simulink model "ex_lateral_dynamics"  (R2026a)
settings: Solver=VariableStepAuto
libraries: aerolibconvert2 x1
settings Model: Creator=doyeop  LastModifiedBy=doyeop

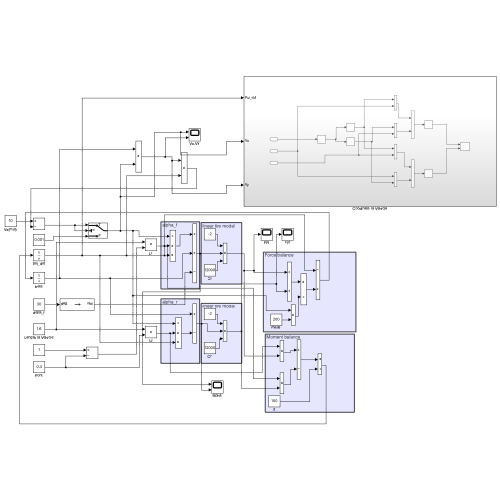
[thumbnail: Simulink's stored preview of the top-level diagram]
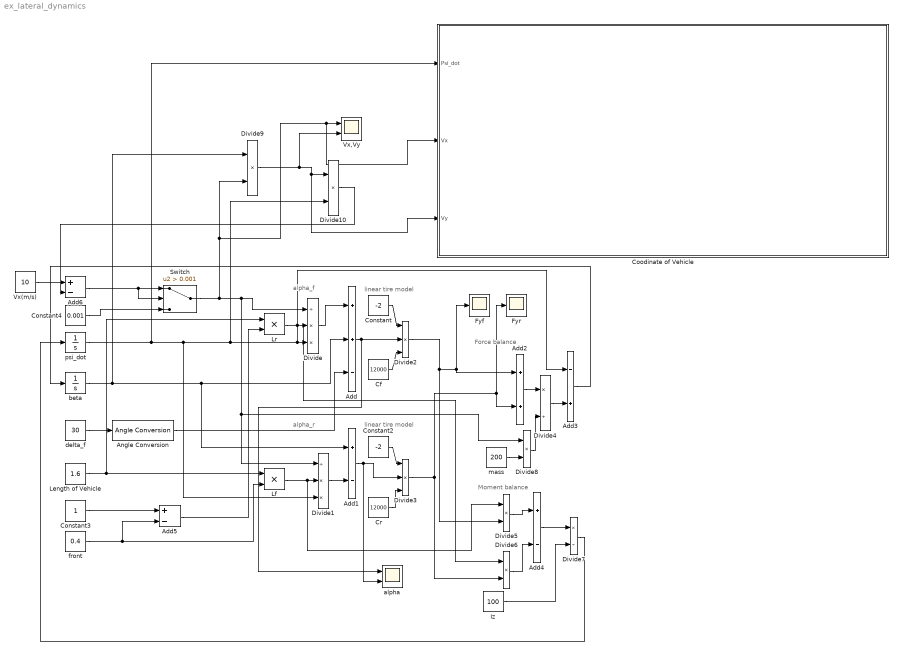
== system ex_lateral_dynamics ==
  note: linear tire model
  note: linear tire model
  note: alpha_f
  note: Moment balance
  note: alpha_r
  note: Force balance
  Add : Sum  Inputs=++-
  Add{1,4..6} (4 alike) : Sum  Inputs=+-
  Add2 : Sum
  Add3 : Sum  Inputs=-+
  Angle Conversion : aerolibconvert2/Angle Conversion  IU=deg  OU=rad
  Cf : Constant  Value=12000  SampleTime=-1
  Constant : Constant  Value=-2  SampleTime=-1
  Constant2 : Constant  Value=-2  SampleTime=-1
  Constant3 : Constant  SampleTime=-1
  Constant4 : Constant  Value=0.001
  Coodinate of Vehicle : Subsystem
  Cr : Constant  Value=12000  SampleTime=-1
  Divide : Product  Inputs=/**
  Divide1 : Product  Inputs=/**
  Divide{5..6,8..10} (5 alike) : Product  Inputs=**
  Divide2 : Product  Inputs=***
  Divide3 : Product  Inputs=***
  Divide4 : Product  Inputs=*/
  Divide7 : Product  Inputs=*/
  Fyf : Scope
      settings: ActiveDisplayYMinimum=-1407.4048741262529  ActiveDisplayYMaximum=11639.532558539519  DataLoggingVariableName=ScopeData14
  Fyr : Scope
      settings: ActiveDisplayYMinimum=-970.12534509010345  ActiveDisplayYMaximum=7745.6964021526865  DataLoggingVariableName=ScopeData15
  Iz : Constant  Value=100  SampleTime=-1
  Length of Vehicle : Constant  Value=1.6
  Lf : Product
  Lr : Product
  Switch : Switch  Criteria=u2 > Threshold  Threshold=0.001  SaturateOnIntegerOverflow=off  InputSameDT=off
  Vx(m/s) : Constant  Value=10
  Vx,Vy : Scope  NumInputPorts=2
      settings: ActiveDisplayYMinimum=-1.2499999999999998  ActiveDisplayYMaximum=11.25  DataLoggingVariableName=ScopeData16
  alpha : Scope  NumInputPorts=2
      settings: ActiveDisplayYMinimum=-0.10159314992994704  ActiveDisplayYMaximum=0.04167372337235864  DataLoggingVariableName=ScopeData27
  beta : Integrator
  delta_f : Constant  Value=30  SampleTime=-1
  front : Constant  Value=0.4  SampleTime=-1
  mass : Constant  Value=200
  psi_dot : Integrator
  wires:
  Cr/1 -> Divide3/3
  Add1/1 -> alpha/2, Divide3/2
  Constant2/1 -> Divide3/1
  Cf/1 -> Divide2/3
  Add3/1 -> beta/1
  Add/1 -> alpha/1, Divide2/2
  Constant/1 -> Divide2/1
  Divide10/1 -> Add6/2
  Angle Conversion/1 -> Add/3
  beta/1 -> Divide9/1, Add1/1, Add/2
  psi_dot/1 -> Add3/1, Divide/3, Divide10/2, Divide1/3, Coodinate of Vehicle/1(Psi_dot)
  Constant4/1 -> Switch/3
  Divide1/1 -> Add1/2
  Iz/1 -> Divide7/2
  Divide8/1 -> Divide4/2
  Switch/1 -> Divide1/1, Divide8/1, Divide/1, Divide9/2, Coodinate of Vehicle/2(Vx), Vx,Vy/1
  Divide/1 -> Add/1
  Divide9/1 -> Coodinate of Vehicle/3(Vy), Divide10/1, Vx,Vy/2
  Divide2/1 -> Divide5/2, Fyf/1, Add2/1
  Divide3/1 -> Add2/2, Fyr/1, Divide6/2
  Add2/1 -> Divide4/1
  delta_f/1 -> Angle Conversion/1
  mass/1 -> Divide8/2
  Divide7/1 -> psi_dot/1
  Add4/1 -> Divide7/1
  Divide6/1 -> Add4/2
  Divide5/1 -> Add4/1
  Divide4/1 -> Add3/2
  Add5/1 -> Lr/2
  Lf/1 -> Divide5/1, Divide1/2
  Lr/1 -> Divide6/1, Divide/2
  front/1 -> Lf/2, Add5/2
  Constant3/1 -> Add5/1
  Length of Vehicle/1 -> Lf/1, Lr/1
  Vx(m/s)/1 -> Add6/1
  Add6/1 -> Switch/2, Switch/1

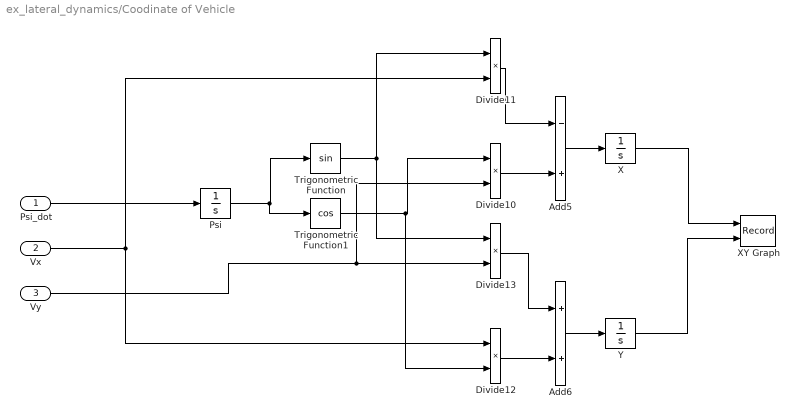
== system ex_lateral_dynamics/Coodinate of Vehicle ==
  Psi_dot : Inport
  Vx : Inport  Port=2
  Vy : Inport  Port=3
  Add5 : Sum  Inputs=-+
  Add6 : Sum
  Divide{10..13} (4 alike) : Product  Inputs=**
  Psi : Integrator
  Trigonometric Function : Trigonometry
  Trigonometric Function1 : Trigonometry  Operator=cos
  X : Integrator
  XY Graph : Record  NumPorts=2.0  FileSettingsInternal="{\"entries\":[{\"content\":{\"excelSettings\":{\"content\":{},\"type\":\"Streamout.ExcelSettings\"},\"parquetSettings\":{\"content\":{},\"type\":\"Streamout.ParquetSettings\"}},\"type\":\"Streamout.FileSettingStorage\",\"uuid\":\"\"}],\"packageUris\":[\"http:\\/\\/schema.mathworks.com\\/mf0\\/streamout_blocks\\/R2020a\"],\"version\":\"1.0\"}"  FrameSettings=[0, 0]  Layout=[1 1]  SignalsInternal="{\"entries\":[{\"content\":{\"signals\":[{\"content\":{\"blockPath\":[],\"dimensions\":[1],\"domain\":\"\",\"lineColor\":\"#a2142f\",\"plots\":[ 1 ],\"port\":1,\"sid\":[\"\"],\"signalID\":1,\"signalName\":\"X\"},\"type\":\"RecordBlkView.Signal\",\"uuid\":\"\"},{\"content\":{\"blockPath\":[],\"dimensions\":[1],\"domain\":\"\",\"lineColor\":\"#139fff\",\"plots\":[ 1 ],\"port\":2,\"sid\":[\"\"],\"signalID\":2,\"signalName\":\"Y\"},\"type\":\"RecordBlkView.Signal\",\"uuid\":\"\"}]},\"type\":\"RecordBlkView.InputSignals\",\"uuid\":\"\"}],\"packageUris\":[\"http:\\/\\/schema.mathworks.com\\/mf0\\/streamout_blocks\\/R2020a\"],\"version\":\"1.0\"}"  VisualizationBindings="{\"xyplotplugin\":{\"info\":[{\"series\":[{\"bindingParametersList\":[{\"parameter\":\"X-Axis\",\"signalID\":1,\"signalName\":\"X\"},{\"parameter\":\"Y-Axis\",\"signalID\":2,\"signalName\":\"Y\"}],\"seriesID\":0}],\"subplotID\":1}]}}"  CompatibilityTag=XY
  Y : Integrator
  wires:
  X/1 -> XY Graph/1
  Add6/1 -> Y/1
  Divide10/1 -> Add5/2
  Psi/1 -> Trigonometric Function1/1, Trigonometric Function/1
  Divide12/1 -> Add6/2
  Trigonometric Function1/1 -> Divide12/2, Divide10/1
  Y/1 -> XY Graph/2
  Divide13/1 -> Add6/1
  Psi_dot/1 -> Psi/1
  Add5/1 -> X/1
  Trigonometric Function/1 -> Divide11/1, Divide13/1
  Divide11/1 -> Add5/1
  Vx/1 -> Divide12/1, Divide11/2
  Vy/1 -> Divide10/2, Divide13/2
